simulink library "wt_blockset_v3"  (Simulink 6.0)
settings: Solver=ode45  SolverMode=SingleTasking  StartTime=0.0  StopTime=10.0  RelTol=1e-3
undefined symbols (not defined in the file): f1, get, j, Kmode, Type, u0
libraries: simulink_extras x12, simulink3 x5, simulink x4, dspinverses x1, dspmtrx3 x1, dspsnks4 x1
(part 7 of 7)

== system wt_blockset_v3/Power Converters/Average SVM Strategy/3rd quadrant/Sector 4 ==
  note: Sector 4
  vd : Inport  Port=1  LatchInput=off
  vq : Inport  Port=2  LatchInput=off
  Action Port : ActionPort  InitializeStates=reset
  Constant : Constant  Value=0.5
  Mux : Mux  Inputs=3
  Mux1 : Mux  Inputs=3
  Mux2 : Mux  Inputs=3
  Mux3 : Mux  Inputs=2
  Sum : Sum  Inputs=-+-  SaturateOnIntegerOverflow=on
  T0_pr : Fcn  Expr=(u(2)<=0)*0+(u(2)>0)*u(2)
  T1_pr : Fcn  Expr=(u(2)<=0)*(0.5*u(1)/(u(1)+u(3)))+(u(2)>0)*u(1)
  T2_pr : Fcn  Expr=(u(2)<=0)*(0.5*u(3)/(u(1)+u(3)))+(u(2)>0)*u(3)
  T_1 : Fcn  Expr=0.5*(-u(1)+abs(u(2))/sqrt(3))
  T_2 : Fcn  Expr=0.5*(u(1)+abs(u(2))/sqrt(3))
  duty_A : Fcn  Expr=1-(u(3)+2*u(1))
  duty_B : Fcn  Expr=u(3)
  duty_C : Fcn  Expr=1-u(3)
  duty_ABC : Outport  OutputWhenDisabled=reset  InitialOutput=[0 0 0]
  wires:
  Sum/1 -> Mux1/2
  Constant/1 -> Sum/2
  T_1/1 -> Sum/1, Mux1/1
  T_2/1 -> Mux1/3, Sum/3
  Mux1/1 -> T1_pr/1, T2_pr/1, T0_pr/1
  T0_pr/1 -> [T0]
  T1_pr/1 -> [T1]
  T2_pr/1 -> [T2]
  [T1] -> Mux2/1
  [T2] -> Mux2/2
  [T0] -> Mux2/3
  Mux/1 -> duty_ABC/1
  Mux2/1 -> duty_A/1, duty_B/1, duty_C/1
  duty_A/1 -> Mux/1
  Mux3/1 -> T_1/1, T_2/1
  vq/1 -> Mux3/2
  vd/1 -> Mux3/1
  duty_B/1 -> Mux/2
  duty_C/1 -> Mux/3

== system wt_blockset_v3/Power Converters/Average SVM Strategy/4th quadrant/Sector 4 ==
  note: Sector 4
  vd : Inport  Port=1  LatchInput=off
  vq : Inport  Port=2  LatchInput=off
  Action Port : ActionPort  InitializeStates=reset
  Constant : Constant  Value=0.5
  Mux : Mux  Inputs=3
  Mux1 : Mux  Inputs=3
  Mux2 : Mux  Inputs=3
  Mux3 : Mux  Inputs=2
  Sum : Sum  Inputs=-+-  SaturateOnIntegerOverflow=on
  T0_pr : Fcn  Expr=(u(2)<=0)*0+(u(2)>0)*u(2)
  T1_pr : Fcn  Expr=(u(2)<=0)*(0.5*u(1)/(u(1)+u(3)))+(u(2)>0)*u(1)
  T2_pr : Fcn  Expr=(u(2)<=0)*(0.5*u(3)/(u(1)+u(3)))+(u(2)>0)*u(3)
  T_1 : Fcn  Expr=0.5*(-u(1)+abs(u(2))/sqrt(3))
  T_2 : Fcn  Expr=0.5*(u(1)+abs(u(2))/sqrt(3))
  duty_A : Fcn  Expr=1-(u(3)+2*u(1))
  duty_B : Fcn  Expr=u(3)
  duty_C : Fcn  Expr=1-u(3)
  duty_ABC : Outport  OutputWhenDisabled=reset  InitialOutput=[0 0 0]
  wires:
  duty_C/1 -> Mux/3
  duty_B/1 -> Mux/2
  vd/1 -> Mux3/1
  vq/1 -> Mux3/2
  Mux3/1 -> T_2/1, T_1/1
  duty_A/1 -> Mux/1
  Mux2/1 -> duty_C/1, duty_B/1, duty_A/1
  Mux/1 -> duty_ABC/1
  [T0] -> Mux2/3
  [T2] -> Mux2/2
  [T1] -> Mux2/1
  T0_pr/1 -> [T0]
  T2_pr/1 -> [T2]
  T1_pr/1 -> [T1]
  Mux1/1 -> T0_pr/1, T2_pr/1, T1_pr/1
  T_2/1 -> Sum/3, Mux1/3
  T_1/1 -> Mux1/1, Sum/1
  Constant/1 -> Sum/2
  Sum/1 -> Mux1/2

== system wt_blockset_v3/Power Converters/Average SVM Strategy/4th quadrant/Sector 5 ==
  note: Sector 5
  vd : Inport  Port=1  LatchInput=off
  vq : Inport  Port=2  LatchInput=off
  Action Port : ActionPort  InitializeStates=reset
  Constant : Constant  Value=0.5
  Mux : Mux  Inputs=3
  Mux1 : Mux  Inputs=3
  Mux2 : Mux  Inputs=3
  Mux3 : Mux  Inputs=2
  Sum : Sum  Inputs=-+-  SaturateOnIntegerOverflow=on
  T0_pr : Fcn  Expr=(u(2)<=0)*0+(u(2)>0)*u(2)
  T1_pr : Fcn  Expr=(u(2)<=0)*(0.5*u(1)/(u(1)+u(3)))+(u(2)>0)*u(1)
  T2_pr : Fcn  Expr=(u(2)<=0)*(0.5*u(3)/(u(1)+u(3)))+(u(2)>0)*u(3)
  T_1 : Fcn  Expr=0.5*((u(1))-abs(u(2))/sqrt(3))
  T_2 : Fcn  Expr=abs(u(2))/sqrt(3)
  duty_A : Fcn  Expr=1-u(3)
  duty_B : Fcn  Expr=u(3)
  duty_C : Fcn  Expr=1-(u(3)+2*u(1))
  duty_ABC : Outport  OutputWhenDisabled=reset  InitialOutput=[0 0 0]
  wires:
  vd/1 -> Mux3/1
  vq/1 -> Mux3/2
  Constant/1 -> Sum/2
  Sum/1 -> Mux1/2
  T1_pr/1 -> [T1]
  T2_pr/1 -> [T2]
  T0_pr/1 -> [T0]
  Mux1/1 -> T1_pr/1, T2_pr/1, T0_pr/1
  [T1] -> Mux2/1
  [T2] -> Mux2/2
  [T0] -> Mux2/3
  Mux/1 -> duty_ABC/1
  T_2/1 -> Mux1/3, Sum/3
  T_1/1 -> Mux1/1, Sum/1
  Mux3/1 -> T_1/1, T_2/1
  duty_A/1 -> Mux/1
  duty_B/1 -> Mux/2
  duty_C/1 -> Mux/3
  Mux2/1 -> duty_B/1, duty_A/1, duty_C/1

== system wt_blockset_v3/Power Converters/Soft-Starter/S-R flip flop/S-R Flip-Flop1 ==
  S : Inport  Port=1  LatchInput=off
  R : Inport  Port=2  LatchInput=off
  Demux : Demux  Outputs=2
  Logic : CombinatorialLogic  TruthTable=[0 1;1 0;0 1;0 1;1 0;1 0;0 0;0 0]
  Memory : Memory  Orientation=left  X0=initial_condition  InheritSampleTime=on
  Mux : Mux  Inputs=3
  Q : Outport  InitialOutput=0
  !Q : Outport  Port=2  InitialOutput=1
  wires:
  Memory/1 -> Mux/3
  Mux/1 -> Logic/1
  Logic/1 -> Demux/1
  Demux/2 -> !Q/1
  Demux/1 -> Q/1, Memory/1
  S/1 -> Mux/1
  R/1 -> Mux/2

== system wt_blockset_v3/Power Converters/Soft-Starter/S-R flip flop/S-R Flip-Flop2 ==
  S : Inport  Port=1  LatchInput=off
  R : Inport  Port=2  LatchInput=off
  Demux : Demux  Outputs=2
  Logic : CombinatorialLogic  TruthTable=[0 1;1 0;0 1;0 1;1 0;1 0;0 0;0 0]
  Memory : Memory  Orientation=left  X0=initial_condition  InheritSampleTime=on
  Mux : Mux  Inputs=3
  Q : Outport  InitialOutput=0
  !Q : Outport  Port=2  InitialOutput=1
  wires:
  Memory/1 -> Mux/3
  Mux/1 -> Logic/1
  Logic/1 -> Demux/1
  Demux/2 -> !Q/1
  Demux/1 -> Q/1, Memory/1
  S/1 -> Mux/1
  R/1 -> Mux/2

== system wt_blockset_v3/Power Converters/Soft-Starter/S-R flip flop/S-R Flip-Flop3 ==
  S : Inport  Port=1  LatchInput=off
  R : Inport  Port=2  LatchInput=off
  Demux : Demux  Outputs=2
  Logic : CombinatorialLogic  TruthTable=[0 1;1 0;0 1;0 1;1 0;1 0;0 0;0 0]
  Memory : Memory  Orientation=left  X0=initial_condition  InheritSampleTime=on
  Mux : Mux  Inputs=3
  Q : Outport  InitialOutput=0
  !Q : Outport  Port=2  InitialOutput=1
  wires:
  Memory/1 -> Mux/3
  Mux/1 -> Logic/1
  Logic/1 -> Demux/1
  Demux/2 -> !Q/1
  Demux/1 -> Q/1, Memory/1
  S/1 -> Mux/1
  R/1 -> Mux/2

== system wt_blockset_v3/Power Converters/Soft-Starter/S-R flip flop/S-R Flip-Flop4 ==
  S : Inport  Port=1  LatchInput=off
  R : Inport  Port=2  LatchInput=off
  Demux : Demux  Outputs=2
  Logic : CombinatorialLogic  TruthTable=[0 1;1 0;0 1;0 1;1 0;1 0;0 0;0 0]
  Memory : Memory  Orientation=left  X0=initial_condition  InheritSampleTime=on
  Mux : Mux  Inputs=3
  Q : Outport  InitialOutput=0
  !Q : Outport  Port=2  InitialOutput=1
  wires:
  Memory/1 -> Mux/3
  Mux/1 -> Logic/1
  Logic/1 -> Demux/1
  Demux/2 -> !Q/1
  Demux/1 -> Q/1, Memory/1
  S/1 -> Mux/1
  R/1 -> Mux/2

== system wt_blockset_v3/Power Converters/Soft-Starter/S-R flip flop/S-R Flip-Flop5 ==
  S : Inport  Port=1  LatchInput=off
  R : Inport  Port=2  LatchInput=off
  Demux : Demux  Outputs=2
  Logic : CombinatorialLogic  TruthTable=[0 1;1 0;0 1;0 1;1 0;1 0;0 0;0 0]
  Memory : Memory  Orientation=left  X0=initial_condition  InheritSampleTime=on
  Mux : Mux  Inputs=3
  Q : Outport  InitialOutput=0
  !Q : Outport  Port=2  InitialOutput=1
  wires:
  Memory/1 -> Mux/3
  Mux/1 -> Logic/1
  Logic/1 -> Demux/1
  Demux/2 -> !Q/1
  Demux/1 -> Q/1, Memory/1
  S/1 -> Mux/1
  R/1 -> Mux/2

== system wt_blockset_v3/Power Converters/Soft-Starter/S-R flip flop/S-R Flip-Flop6 ==
  S : Inport  Port=1  LatchInput=off
  R : Inport  Port=2  LatchInput=off
  Demux : Demux  Outputs=2
  Logic : CombinatorialLogic  TruthTable=[0 1;1 0;0 1;0 1;1 0;1 0;0 0;0 0]
  Memory : Memory  Orientation=left  X0=initial_condition  InheritSampleTime=on
  Mux : Mux  Inputs=3
  Q : Outport  InitialOutput=0
  !Q : Outport  Port=2  InitialOutput=1
  wires:
  Memory/1 -> Mux/3
  Mux/1 -> Logic/1
  Logic/1 -> Demux/1
  Demux/2 -> !Q/1
  Demux/1 -> Q/1, Memory/1
  S/1 -> Mux/1
  R/1 -> Mux/2

== system wt_blockset_v3/Power Converters/Soft-Starter/S-R flip flop1/S-R Flip-Flop1 ==
  S : Inport  Port=1  LatchInput=off
  R : Inport  Port=2  LatchInput=off
  Demux : Demux  Outputs=2
  Logic : CombinatorialLogic  TruthTable=[0 1;1 0;0 1;0 1;1 0;1 0;0 0;0 0]
  Memory : Memory  Orientation=left  X0=initial_condition  InheritSampleTime=on
  Mux : Mux  Inputs=3
  Q : Outport  InitialOutput=0
  !Q : Outport  Port=2  InitialOutput=1
  wires:
  R/1 -> Mux/2
  S/1 -> Mux/1
  Demux/1 -> Memory/1, Q/1
  Demux/2 -> !Q/1
  Logic/1 -> Demux/1
  Mux/1 -> Logic/1
  Memory/1 -> Mux/3

== system wt_blockset_v3/Power Converters/Soft-Starter/S-R flip flop1/S-R Flip-Flop2 ==
  S : Inport  Port=1  LatchInput=off
  R : Inport  Port=2  LatchInput=off
  Demux : Demux  Outputs=2
  Logic : CombinatorialLogic  TruthTable=[0 1;1 0;0 1;0 1;1 0;1 0;0 0;0 0]
  Memory : Memory  Orientation=left  X0=initial_condition  InheritSampleTime=on
  Mux : Mux  Inputs=3
  Q : Outport  InitialOutput=0
  !Q : Outport  Port=2  InitialOutput=1
  wires:
  Memory/1 -> Mux/3
  Mux/1 -> Logic/1
  Logic/1 -> Demux/1
  Demux/2 -> !Q/1
  Demux/1 -> Q/1, Memory/1
  S/1 -> Mux/1
  R/1 -> Mux/2

== system wt_blockset_v3/Power Converters/Soft-Starter/S-R flip flop1/S-R Flip-Flop3 ==
  S : Inport  Port=1  LatchInput=off
  R : Inport  Port=2  LatchInput=off
  Demux : Demux  Outputs=2
  Logic : CombinatorialLogic  TruthTable=[0 1;1 0;0 1;0 1;1 0;1 0;0 0;0 0]
  Memory : Memory  Orientation=left  X0=initial_condition  InheritSampleTime=on
  Mux : Mux  Inputs=3
  Q : Outport  InitialOutput=0
  !Q : Outport  Port=2  InitialOutput=1
  wires:
  Memory/1 -> Mux/3
  Mux/1 -> Logic/1
  Logic/1 -> Demux/1
  Demux/2 -> !Q/1
  Demux/1 -> Q/1, Memory/1
  S/1 -> Mux/1
  R/1 -> Mux/2

== system wt_blockset_v3/Power Converters/Soft-Starter/S-R flip flop1/S-R Flip-Flop4 ==
  S : Inport  Port=1  LatchInput=off
  R : Inport  Port=2  LatchInput=off
  Demux : Demux  Outputs=2
  Logic : CombinatorialLogic  TruthTable=[0 1;1 0;0 1;0 1;1 0;1 0;0 0;0 0]
  Memory : Memory  Orientation=left  X0=initial_condition  InheritSampleTime=on
  Mux : Mux  Inputs=3
  Q : Outport  InitialOutput=0
  !Q : Outport  Port=2  InitialOutput=1
  wires:
  Memory/1 -> Mux/3
  Mux/1 -> Logic/1
  Logic/1 -> Demux/1
  Demux/2 -> !Q/1
  Demux/1 -> Q/1, Memory/1
  S/1 -> Mux/1
  R/1 -> Mux/2

== system wt_blockset_v3/Power Converters/Soft-Starter/S-R flip flop1/S-R Flip-Flop5 ==
  S : Inport  Port=1  LatchInput=off
  R : Inport  Port=2  LatchInput=off
  Demux : Demux  Outputs=2
  Logic : CombinatorialLogic  TruthTable=[0 1;1 0;0 1;0 1;1 0;1 0;0 0;0 0]
  Memory : Memory  Orientation=left  X0=initial_condition  InheritSampleTime=on
  Mux : Mux  Inputs=3
  Q : Outport  InitialOutput=0
  !Q : Outport  Port=2  InitialOutput=1
  wires:
  Memory/1 -> Mux/3
  Mux/1 -> Logic/1
  Logic/1 -> Demux/1
  Demux/2 -> !Q/1
  Demux/1 -> Q/1, Memory/1
  S/1 -> Mux/1
  R/1 -> Mux/2

== system wt_blockset_v3/Power Converters/Soft-Starter/S-R flip flop1/S-R Flip-Flop6 ==
  S : Inport  Port=1  LatchInput=off
  R : Inport  Port=2  LatchInput=off
  Demux : Demux  Outputs=2
  Logic : CombinatorialLogic  TruthTable=[0 1;1 0;0 1;0 1;1 0;1 0;0 0;0 0]
  Memory : Memory  Orientation=left  X0=initial_condition  InheritSampleTime=on
  Mux : Mux  Inputs=3
  Q : Outport  InitialOutput=0
  !Q : Outport  Port=2  InitialOutput=1
  wires:
  Memory/1 -> Mux/3
  Mux/1 -> Logic/1
  Logic/1 -> Demux/1
  Demux/2 -> !Q/1
  Demux/1 -> Q/1, Memory/1
  S/1 -> Mux/1
  R/1 -> Mux/2

== system wt_blockset_v3/Power Converters/Switching PWM Strategy/capcom/Vtri1 ==
  Constant1 : Constant
  Constant2 : Constant
  Constant3 : Constant  Value=0
  Data Type Conversion : DataTypeConversion  SaturateOnIntegerOverflow=on  RndMeth=Zero
  Fcn : Fcn  Expr=-u(1)*2+1
  Gain : Gain  Gain=fsw2  SaturateOnIntegerOverflow=on
  Gain1 : Gain  Gain=2*fsw2  SaturateOnIntegerOverflow=on
  IC : InitialCondition  Value=1.5
  Integrator : Integrator  ExternalReset=rising  InitialConditionSource=external  InitialCondition=1.5
  Integrator1 : Integrator  ExternalReset=rising
  Pulse Generator : DiscretePulseGenerator  PulseType=Time based  Period=2/fsw2  PulseWidth=50  PhaseDelay=0.5/fsw2
  Pulse Generator1 : DiscretePulseGenerator  PulseType=Time based  Period=2/fsw2  PulseWidth=50
  Relational Operator : RelationalOperator  InputSameDT=on
  Vtri : Outport  InitialOutput=0
  wires:
  Integrator1/1 -> Vtri/1
  Pulse Generator/1 -> Integrator/2
  Constant2/1 -> Gain/1
  Fcn/1 -> Gain1/1
  Relational Operator/1 -> Data Type Conversion/1
  Integrator/1 -> Relational Operator/1
  IC/1 -> Integrator/3
  Constant3/1 -> IC/1
  Pulse Generator1/1 -> Integrator1/2
  Gain1/1 -> Integrator1/1
  Gain/1 -> Integrator/1
  Constant1/1 -> Relational Operator/2
  Data Type Conversion/1 -> Fcn/1

== system wt_blockset_v3/Power Converters/Switching PWM Strategy/capcom/pulses ==
  In1 : Inport  Port=1  LatchInput=off
  Constant : Constant  Value=0
  Data Type Conversion : DataTypeConversion  OutDataTypeMode=double  SaturateOnIntegerOverflow=on  RndMeth=Zero
  Hit  Crossing : HitCross  ShowOutputPort=off
  IC : InitialCondition  Value=0
  Relational Operator : RelationalOperator  InputSameDT=on
  Out1 : Outport  InitialOutput=0
  wires:
  Relational Operator/1 -> Data Type Conversion/1
  In1/1 -> Relational Operator/1
  Constant/1 -> Relational Operator/2
  IC/1 -> Out1/1
  Data Type Conversion/1 -> Hit  Crossing/1, IC/1

== system wt_blockset_v3/Power Converters/Switching SVM Strategy/1st quadrant/Sector 0 ==
  note: Sector 0
  vd : Inport  Port=1  LatchInput=off
  vq : Inport  Port=2  LatchInput=off
  Action Port : ActionPort  InitializeStates=reset
  Constant : Constant  Value=0.5
  Mux : Mux  Inputs=3
  Mux1 : Mux  Inputs=3
  Mux2 : Mux  Inputs=3
  Mux3 : Mux  Inputs=2
  Sum : Sum  Inputs=-+-  SaturateOnIntegerOverflow=on
  T0_pr : Fcn  Expr=(u(2)<=0)*0+(u(2)>0)*u(2)
  T1_pr : Fcn  Expr=(u(2)<=0)*(0.5*u(1)/(u(1)+u(3)))+(u(2)>0)*u(1)
  T2_pr : Fcn  Expr=(u(2)<=0)*(0.5*u(3)/(u(1)+u(3)))+(u(2)>0)*u(3)
  T_1 : Fcn  Expr=0.5*(u(1)-u(2)/sqrt(3))
  T_2 : Fcn  Expr=u(2)/sqrt(3)
  duty_A : Fcn  Expr=1-u(3)
  duty_B : Fcn  Expr=1-(u(3)+2*u(1))
  duty_C : Fcn  Expr=u(3)
  duty_ABC : Outport  OutputWhenDisabled=reset  InitialOutput=[0 0 0]
  wires:
  T_2/1 -> Sum/3, Mux1/3
  T_1/1 -> Sum/1, Mux1/1
  Constant/1 -> Sum/2
  Sum/1 -> Mux1/2
  T1_pr/1 -> [T1]
  T2_pr/1 -> [T2]
  T0_pr/1 -> [T0]
  Mux1/1 -> T1_pr/1, T2_pr/1, T0_pr/1
  [T1] -> Mux2/1
  [T2] -> Mux2/2
  [T0] -> Mux2/3
  Mux2/1 -> duty_B/1, duty_A/1, duty_C/1
  duty_A/1 -> Mux/1
  duty_B/1 -> Mux/2
  duty_C/1 -> Mux/3
  Mux/1 -> duty_ABC/1
  Mux3/1 -> T_1/1, T_2/1
  vd/1 -> Mux3/1
  vq/1 -> Mux3/2

== system wt_blockset_v3/Power Converters/Switching SVM Strategy/1st quadrant/Sector 1 ==
  note: Sector 1
  vd : Inport  Port=1  LatchInput=off
  vq : Inport  Port=2  LatchInput=off
  Action Port : ActionPort  InitializeStates=reset
  Constant : Constant  Value=0.5
  Mux : Mux  Inputs=3
  Mux1 : Mux  Inputs=3
  Mux2 : Mux  Inputs=3
  Mux3 : Mux  Inputs=2
  Sum : Sum  Inputs=-+-  SaturateOnIntegerOverflow=on
  T0_pr : Fcn  Expr=(u(2)<=0)*0+(u(2)>0)*u(2)
  T1_pr : Fcn  Expr=(u(2)<=0)*(0.5*u(1)/(u(1)+u(3)))+(u(2)>0)*u(1)
  T2_pr : Fcn  Expr=(u(2)<=0)*(0.5*u(3)/(u(1)+u(3)))+(u(2)>0)*u(3)
  T_1 : Fcn  Expr=0.5*(-u(1)+u(2)/sqrt(3))
  T_2 : Fcn  Expr=0.5*(+u(1)+u(2)/sqrt(3))
  duty_A : Fcn  Expr=1-(u(3)+2*u(1))
  duty_B : Fcn  Expr=1-u(3)
  duty_C : Fcn  Expr=u(3)
  duty_ABC : Outport  OutputWhenDisabled=reset  InitialOutput=[0 0 0]
  wires:
  Sum/1 -> Mux1/2
  Constant/1 -> Sum/2
  T_1/1 -> Sum/1, Mux1/1
  T_2/1 -> Mux1/3, Sum/3
  Mux1/1 -> T1_pr/1, T2_pr/1, T0_pr/1
  [T1] -> Mux2/1
  [T2] -> Mux2/2
  [T0] -> Mux2/3
  Mux/1 -> duty_ABC/1
  Mux2/1 -> duty_B/1, duty_A/1, duty_C/1
  duty_B/1 -> Mux/2
  duty_A/1 -> Mux/1
  duty_C/1 -> Mux/3
  Mux3/1 -> T_1/1, T_2/1
  vq/1 -> Mux3/2
  vd/1 -> Mux3/1
  T1_pr/1 -> [T1]
  T2_pr/1 -> [T2]
  T0_pr/1 -> [T0]

== system wt_blockset_v3/Power Converters/Switching SVM Strategy/2nd quadrant/Sector 1 ==
  note: Sector 1
  vd : Inport  Port=1  LatchInput=off
  vq : Inport  Port=2  LatchInput=off
  Action Port : ActionPort  InitializeStates=reset
  Constant : Constant  Value=0.5
  Mux : Mux  Inputs=3
  Mux1 : Mux  Inputs=3
  Mux2 : Mux  Inputs=3
  Mux3 : Mux  Inputs=2
  Sum : Sum  Inputs=-+-  SaturateOnIntegerOverflow=on
  T0_pr : Fcn  Expr=(u(2)<=0)*0+(u(2)>0)*u(2)
  T1_pr : Fcn  Expr=(u(2)<=0)*(0.5*u(1)/(u(1)+u(3)))+(u(2)>0)*u(1)
  T2_pr : Fcn  Expr=(u(2)<=0)*(0.5*u(3)/(u(1)+u(3)))+(u(2)>0)*u(3)
  T_1 : Fcn  Expr=0.5*(-u(1)+u(2)/sqrt(3))
  T_2 : Fcn  Expr=0.5*(+u(1)+u(2)/sqrt(3))
  duty_A : Fcn  Expr=1-(u(3)+2*u(1))
  duty_B : Fcn  Expr=1-u(3)
  duty_C : Fcn  Expr=u(3)
  duty_ABC : Outport  OutputWhenDisabled=reset  InitialOutput=[0 0 0]
  wires:
  Sum/1 -> Mux1/2
  Constant/1 -> Sum/2
  T_1/1 -> Sum/1, Mux1/1
  T_2/1 -> Mux1/3, Sum/3
  Mux1/1 -> T1_pr/1, T2_pr/1, T0_pr/1
  [T1] -> Mux2/1
  [T2] -> Mux2/2
  [T0] -> Mux2/3
  Mux/1 -> duty_ABC/1
  Mux2/1 -> duty_B/1, duty_A/1, duty_C/1
  duty_B/1 -> Mux/2
  duty_A/1 -> Mux/1
  duty_C/1 -> Mux/3
  Mux3/1 -> T_1/1, T_2/1
  vq/1 -> Mux3/2
  vd/1 -> Mux3/1
  T1_pr/1 -> [T1]
  T2_pr/1 -> [T2]
  T0_pr/1 -> [T0]

== system wt_blockset_v3/Power Converters/Switching SVM Strategy/2nd quadrant/Sector 2 ==
  note: Sector 2
  vd : Inport  Port=1  LatchInput=off
  vq : Inport  Port=2  LatchInput=off
  Action Port : ActionPort  InitializeStates=reset
  Constant : Constant  Value=0.5
  Mux : Mux  Inputs=3
  Mux1 : Mux  Inputs=3
  Mux2 : Mux  Inputs=3
  Mux3 : Mux  Inputs=2
  Sum : Sum  Inputs=-+-  SaturateOnIntegerOverflow=on
  T0_pr : Fcn  Expr=(u(2)<=0)*0+(u(2)>0)*u(2)
  T1_pr : Fcn  Expr=(u(2)<=0)*(0.5*u(1)/(u(1)+u(3)))+(u(2)>0)*u(1)
  T2_pr : Fcn  Expr=(u(2)<=0)*(0.5*u(3)/(u(1)+u(3)))+(u(2)>0)*u(3)
  T_ : Fcn  Expr=0.5*(abs(u(1))-u(2)/sqrt(3))
  T_1 : Fcn  Expr=u(2)/sqrt(3)
  duty_A : Fcn  Expr=u(3)
  duty_B : Fcn  Expr=1-u(3)
  duty_C : Fcn  Expr=1-(u(3)+2*u(1))
  duty_ABC : Outport  OutputWhenDisabled=reset  InitialOutput=[0 0 0]
  wires:
  Mux/1 -> duty_ABC/1
  [T0] -> Mux2/3
  [T2] -> Mux2/2
  [T1] -> Mux2/1
  Mux1/1 -> T0_pr/1, T2_pr/1, T1_pr/1
  Sum/1 -> Mux1/2
  Constant/1 -> Sum/2
  vq/1 -> Mux3/2
  vd/1 -> Mux3/1
  Mux3/1 -> T_1/1, T_/1
  T_1/1 -> Mux1/1, Sum/1
  T_/1 -> Mux1/3, Sum/3
  duty_B/1 -> Mux/2
  duty_A/1 -> Mux/1
  duty_C/1 -> Mux/3
  Mux2/1 -> duty_B/1, duty_A/1, duty_C/1
  T1_pr/1 -> [T1]
  T2_pr/1 -> [T2]
  T0_pr/1 -> [T0]

== system wt_blockset_v3/Power Converters/Switching SVM Strategy/3rd quadrant/Sector 3 ==
  note: Sector 2
  vd : Inport  Port=1  LatchInput=off
  vq : Inport  Port=2  LatchInput=off
  Action Port : ActionPort  InitializeStates=reset
  Constant : Constant  Value=0.5
  Mux : Mux  Inputs=3
  Mux1 : Mux  Inputs=3
  Mux2 : Mux  Inputs=3
  Mux3 : Mux  Inputs=2
  Sum : Sum  Inputs=-+-  SaturateOnIntegerOverflow=on
  T0_pr : Fcn  Expr=(u(2)<=0)*0+(u(2)>0)*u(2)
  T1_pr : Fcn  Expr=(u(2)<=0)*(0.5*u(1)/(u(1)+u(3)))+(u(2)>0)*u(1)
  T2_pr : Fcn  Expr=(u(2)<=0)*(0.5*u(3)/(u(1)+u(3)))+(u(2)>0)*u(3)
  T_ : Fcn  Expr=0.5*(abs(u(1))-abs(u(2))/sqrt(3))
  T_1 : Fcn  Expr=abs(u(2))/sqrt(3)
  duty_A : Fcn  Expr=u(3)
  duty_B : Fcn  Expr=1-(u(3)+2*u(1))
  duty_C : Fcn  Expr=1-u(3)
  duty_ABC : Outport  OutputWhenDisabled=reset  InitialOutput=[0 0 0]
  wires:
  Mux/1 -> duty_ABC/1
  [T0] -> Mux2/3
  [T2] -> Mux2/2
  [T1] -> Mux2/1
  Mux1/1 -> T0_pr/1, T2_pr/1, T1_pr/1
  Sum/1 -> Mux1/2
  Constant/1 -> Sum/2
  vq/1 -> Mux3/2
  vd/1 -> Mux3/1
  Mux3/1 -> T_1/1, T_/1
  T_1/1 -> Mux1/1, Sum/1
  T_/1 -> Mux1/3, Sum/3
  duty_A/1 -> Mux/1
  Mux2/1 -> duty_A/1, duty_B/1, duty_C/1
  duty_B/1 -> Mux/2
  duty_C/1 -> Mux/3
  T1_pr/1 -> [T1]
  T2_pr/1 -> [T2]
  T0_pr/1 -> [T0]

== system wt_blockset_v3/Power Converters/Switching SVM Strategy/3rd quadrant/Sector 4 ==
  note: Sector 4
  vd : Inport  Port=1  LatchInput=off
  vq : Inport  Port=2  LatchInput=off
  Action Port : ActionPort  InitializeStates=reset
  Constant : Constant  Value=0.5
  Mux : Mux  Inputs=3
  Mux1 : Mux  Inputs=3
  Mux2 : Mux  Inputs=3
  Mux3 : Mux  Inputs=2
  Sum : Sum  Inputs=-+-  SaturateOnIntegerOverflow=on
  T0_pr : Fcn  Expr=(u(2)<=0)*0+(u(2)>0)*u(2)
  T1_pr : Fcn  Expr=(u(2)<=0)*(0.5*u(1)/(u(1)+u(3)))+(u(2)>0)*u(1)
  T2_pr : Fcn  Expr=(u(2)<=0)*(0.5*u(3)/(u(1)+u(3)))+(u(2)>0)*u(3)
  T_1 : Fcn  Expr=0.5*(-u(1)+abs(u(2))/sqrt(3))
  T_2 : Fcn  Expr=0.5*(u(1)+abs(u(2))/sqrt(3))
  duty_A : Fcn  Expr=1-(u(3)+2*u(1))
  duty_B : Fcn  Expr=u(3)
  duty_C : Fcn  Expr=1-u(3)
  duty_ABC : Outport  OutputWhenDisabled=reset  InitialOutput=[0 0 0]
  wires:
  Sum/1 -> Mux1/2
  Constant/1 -> Sum/2
  T_1/1 -> Sum/1, Mux1/1
  T_2/1 -> Mux1/3, Sum/3
  Mux1/1 -> T1_pr/1, T2_pr/1, T0_pr/1
  [T1] -> Mux2/1
  [T2] -> Mux2/2
  [T0] -> Mux2/3
  Mux/1 -> duty_ABC/1
  Mux2/1 -> duty_A/1, duty_B/1, duty_C/1
  duty_A/1 -> Mux/1
  Mux3/1 -> T_1/1, T_2/1
  vq/1 -> Mux3/2
  vd/1 -> Mux3/1
  duty_B/1 -> Mux/2
  duty_C/1 -> Mux/3
  T1_pr/1 -> [T1]
  T2_pr/1 -> [T2]
  T0_pr/1 -> [T0]

== system wt_blockset_v3/Power Converters/Switching SVM Strategy/4th quadrant/Sector 4 ==
  note: Sector 4
  vd : Inport  Port=1  LatchInput=off
  vq : Inport  Port=2  LatchInput=off
  Action Port : ActionPort  InitializeStates=reset
  Constant : Constant  Value=0.5
  Mux : Mux  Inputs=3
  Mux1 : Mux  Inputs=3
  Mux2 : Mux  Inputs=3
  Mux3 : Mux  Inputs=2
  Sum : Sum  Inputs=-+-  SaturateOnIntegerOverflow=on
  T0_pr : Fcn  Expr=(u(2)<=0)*0+(u(2)>0)*u(2)
  T1_pr : Fcn  Expr=(u(2)<=0)*(0.5*u(1)/(u(1)+u(3)))+(u(2)>0)*u(1)
  T2_pr : Fcn  Expr=(u(2)<=0)*(0.5*u(3)/(u(1)+u(3)))+(u(2)>0)*u(3)
  T_1 : Fcn  Expr=0.5*(-u(1)+abs(u(2))/sqrt(3))
  T_2 : Fcn  Expr=0.5*(u(1)+abs(u(2))/sqrt(3))
  duty_A : Fcn  Expr=1-(u(3)+2*u(1))
  duty_B : Fcn  Expr=u(3)
  duty_C : Fcn  Expr=1-u(3)
  duty_ABC : Outport  OutputWhenDisabled=reset  InitialOutput=[0 0 0]
  wires:
  duty_C/1 -> Mux/3
  duty_B/1 -> Mux/2
  vd/1 -> Mux3/1
  vq/1 -> Mux3/2
  Mux3/1 -> T_2/1, T_1/1
  duty_A/1 -> Mux/1
  Mux2/1 -> duty_C/1, duty_B/1, duty_A/1
  Mux/1 -> duty_ABC/1
  [T0] -> Mux2/3
  [T2] -> Mux2/2
  [T1] -> Mux2/1
  Mux1/1 -> T0_pr/1, T2_pr/1, T1_pr/1
  T_2/1 -> Sum/3, Mux1/3
  T_1/1 -> Mux1/1, Sum/1
  Constant/1 -> Sum/2
  Sum/1 -> Mux1/2
  T1_pr/1 -> [T1]
  T2_pr/1 -> [T2]
  T0_pr/1 -> [T0]

== system wt_blockset_v3/Power Converters/Switching SVM Strategy/4th quadrant/Sector 5 ==
  note: Sector 5
  vd : Inport  Port=1  LatchInput=off
  vq : Inport  Port=2  LatchInput=off
  Action Port : ActionPort  InitializeStates=reset
  Constant : Constant  Value=0.5
  Mux : Mux  Inputs=3
  Mux1 : Mux  Inputs=3
  Mux2 : Mux  Inputs=3
  Mux3 : Mux  Inputs=2
  Sum : Sum  Inputs=-+-  SaturateOnIntegerOverflow=on
  T0_pr : Fcn  Expr=(u(2)<=0)*0+(u(2)>0)*u(2)
  T1_pr : Fcn  Expr=(u(2)<=0)*(0.5*u(1)/(u(1)+u(3)))+(u(2)>0)*u(1)
  T2_pr : Fcn  Expr=(u(2)<=0)*(0.5*u(3)/(u(1)+u(3)))+(u(2)>0)*u(3)
  T_1 : Fcn  Expr=0.5*((u(1))-abs(u(2))/sqrt(3))
  T_2 : Fcn  Expr=abs(u(2))/sqrt(3)
  duty_A : Fcn  Expr=1-u(3)
  duty_B : Fcn  Expr=u(3)
  duty_C : Fcn  Expr=1-(u(3)+2*u(1))
  duty_ABC : Outport  OutputWhenDisabled=reset  InitialOutput=[0 0 0]
  wires:
  vd/1 -> Mux3/1
  vq/1 -> Mux3/2
  Constant/1 -> Sum/2
  Sum/1 -> Mux1/2
  Mux1/1 -> T1_pr/1, T2_pr/1, T0_pr/1
  [T1] -> Mux2/1
  [T2] -> Mux2/2
  [T0] -> Mux2/3
  Mux/1 -> duty_ABC/1
  T_2/1 -> Mux1/3, Sum/3
  T_1/1 -> Mux1/1, Sum/1
  Mux3/1 -> T_1/1, T_2/1
  duty_A/1 -> Mux/1
  duty_B/1 -> Mux/2
  duty_C/1 -> Mux/3
  Mux2/1 -> duty_B/1, duty_A/1, duty_C/1
  T1_pr/1 -> [T1]
  T2_pr/1 -> [T2]
  T0_pr/1 -> [T0]

== system wt_blockset_v3/Electrical Machinery/Simulink Blocks  based Models/Permanent Magnet Synchronous Machine with iron losses/PMSM d-q/Iron losses resistance ==
  wr : Inport  Port=1  LatchInput=off
  Iron losses resistance : Fcn  Expr=0.0329*u[1] /(2*pi)+0.827
  Ri : Outport
  wires:
  wr/1 -> Iron losses resistance/1
  Iron losses resistance/1 -> Ri/1

== system wt_blockset_v3/Electrical Machinery/Simulink Blocks  based Models/Salient-Pole Synchronous Machine constant parameters/Mathematical model/dq / abc ==
  D : Inport  Port=1  LatchInput=off
  Q : Inport  Port=2  LatchInput=off
  theta : Inport  Port=3  LatchInput=off
  Mux : Mux  Inputs=3
  va : Fcn  Expr=u[1]*cos(u[3])-u[2]*sin(u[3])
  vb : Fcn  Expr=u[1]*cos(u[3]-2*pi/3)-u[2]*sin(u[3]-2*pi/3)
  vc : Fcn  Expr=u[1]*cos(u[3]+2*pi/3)-u[2]*sin(u[3]+2*pi/3)
  A : Outport  InitialOutput=0
  B : Outport  Port=2  InitialOutput=0
  C : Outport  Port=3  InitialOutput=0
  wires:
  va/1 -> A/1
  vb/1 -> B/1
  vc/1 -> C/1
  Mux/1 -> va/1, vb/1, vc/1
  D/1 -> Mux/1
  Q/1 -> Mux/2
  theta/1 -> Mux/3

== system wt_blockset_v3/Mechanical Components/Wind Model SB-2/3rd_Harmonic_Filter1/3rd harmonic Filter/Coefficients ==
  avg_wind : Inport  Port=1  LatchInput=off
  BD coeff : Fcn  Expr=0.2766/0.3691/(r/u(1))
  CD coeff : Fcn  Expr=0.0307/0.3691/(r/u(1))^2
  ED coeff : Fcn  Expr=1.7722/0.3691/(r/u(1))
  FD coeff : Fcn  Expr=1/0.3691/(r/u(1))^2
  BD : Outport
  CD : Outport  Port=2
  ED : Outport  Port=3
  FD : Outport  Port=4
  wires:
  avg_wind/1 -> BD coeff/1, CD coeff/1, ED coeff/1, FD coeff/1
  BD coeff/1 -> BD/1
  CD coeff/1 -> CD/1
  ED coeff/1 -> ED/1
  FD coeff/1 -> FD/1

== system wt_blockset_v3/Mechanical Components/Wind Model SB-2/3rd_Harmonic_Filter2/3rd harmonic Filter/Coefficients ==
  avg_wind : Inport  Port=1  LatchInput=off
  BD coeff : Fcn  Expr=0.2766/0.3691/(r/u(1))
  CD coeff : Fcn  Expr=0.0307/0.3691/(r/u(1))^2
  ED coeff : Fcn  Expr=1.7722/0.3691/(r/u(1))
  FD coeff : Fcn  Expr=1/0.3691/(r/u(1))^2
  BD : Outport
  CD : Outport  Port=2
  ED : Outport  Port=3
  FD : Outport  Port=4
  wires:
  FD coeff/1 -> FD/1
  ED coeff/1 -> ED/1
  CD coeff/1 -> CD/1
  BD coeff/1 -> BD/1
  avg_wind/1 -> FD coeff/1, ED coeff/1, CD coeff/1, BD coeff/1

== system wt_blockset_v3/Mechanical Components/Wind Model SB-2/Kaimal_Filter_1/Kaimal Filter/Coefficients ==
  avg_wind : Inport  Port=1  LatchInput=off
  BD coeff : Fcn  Expr=1.3653/1.3463/(L/2/pi/u(1))
  CD coeff : Fcn  Expr=0.9846/1.3463/(L/2/pi/u(1))^2
  ED coeff : Fcn  Expr=3.7593/1.3463/(L/2/pi/u(1))
  FD coeff : Fcn  Expr=1/1.3463/(L/2/pi/u(1))^2
  BD : Outport
  CD : Outport  Port=2
  ED : Outport  Port=3
  FD : Outport  Port=4
  wires:
  avg_wind/1 -> BD coeff/1, CD coeff/1, ED coeff/1, FD coeff/1
  BD coeff/1 -> BD/1
  CD coeff/1 -> CD/1
  ED coeff/1 -> ED/1
  FD coeff/1 -> FD/1

== system wt_blockset_v3/Mechanical Components/Wind Model SB-2/Kaimal_Filter_2/Kaimal Filter/Coefficients ==
  avg_wind : Inport  Port=1  LatchInput=off
  BD coeff : Fcn  Expr=1.3653/1.3463/(L/2/pi/u(1))
  CD coeff : Fcn  Expr=0.9846/1.3463/(L/2/pi/u(1))^2
  ED coeff : Fcn  Expr=3.7593/1.3463/(L/2/pi/u(1))
  FD coeff : Fcn  Expr=1/1.3463/(L/2/pi/u(1))^2
  BD : Outport
  CD : Outport  Port=2
  ED : Outport  Port=3
  FD : Outport  Port=4
  wires:
  FD coeff/1 -> FD/1
  ED coeff/1 -> ED/1
  CD coeff/1 -> CD/1
  BD coeff/1 -> BD/1
  avg_wind/1 -> FD coeff/1, ED coeff/1, CD coeff/1, BD coeff/1

== system wt_blockset_v3/Mechanical Components/Wind Model SB-2/Kaimal_Filter_3/Kaimal Filter/Coefficients ==
  avg_wind : Inport  Port=1  LatchInput=off
  BD coeff : Fcn  Expr=1.3653/1.3463/(L/2/pi/u(1))
  CD coeff : Fcn  Expr=0.9846/1.3463/(L/2/pi/u(1))^2
  ED coeff : Fcn  Expr=3.7593/1.3463/(L/2/pi/u(1))
  FD coeff : Fcn  Expr=1/1.3463/(L/2/pi/u(1))^2
  BD : Outport
  CD : Outport  Port=2
  ED : Outport  Port=3
  FD : Outport  Port=4
  wires:
  avg_wind/1 -> BD coeff/1, CD coeff/1, ED coeff/1, FD coeff/1
  BD coeff/1 -> BD/1
  CD coeff/1 -> CD/1
  ED coeff/1 -> ED/1
  FD coeff/1 -> FD/1

== system wt_blockset_v3/Mechanical Components/Wind Model SB-2/ZERO_Harmonic_Filter/ZERO harmonic Filter/Coefficients ==
  avg_wind : Inport  Port=1  LatchInput=off
  BD coeff : Fcn  Expr=4.7869/7.6823/(r/u(1))
  CD coeff : Fcn  Expr=0.9904/7.6823/(r/u(1))^2
  ED coeff : Fcn  Expr=7.3518/7.6823/(r/u(1))
  FD coeff : Fcn  Expr=1/7.6823/(r/u(1))^2
  BD : Outport
  CD : Outport  Port=2
  ED : Outport  Port=3
  FD : Outport  Port=4
  wires:
  FD coeff/1 -> FD/1
  ED coeff/1 -> ED/1
  CD coeff/1 -> CD/1
  BD coeff/1 -> BD/1
  avg_wind/1 -> FD coeff/1, ED coeff/1, CD coeff/1, BD coeff/1

== system wt_blockset_v3/Mechanical Components/Wind Model ZA-2/3rd_Harmonic_Filter1/3rd harmonic Filter/Coefficients ==
  avg_wind : Inport  Port=1  LatchInput=off
  BD coeff : Fcn  Expr=0.2766/0.3691/(r/u(1))
  CD coeff : Fcn  Expr=0.0307/0.3691/(r/u(1))^2
  ED coeff : Fcn  Expr=1.7722/0.3691/(r/u(1))
  FD coeff : Fcn  Expr=1/0.3691/(r/u(1))^2
  BD : Outport
  CD : Outport  Port=2
  ED : Outport  Port=3
  FD : Outport  Port=4
  wires:
  avg_wind/1 -> BD coeff/1, CD coeff/1, ED coeff/1, FD coeff/1
  BD coeff/1 -> BD/1
  CD coeff/1 -> CD/1
  ED coeff/1 -> ED/1
  FD coeff/1 -> FD/1

== system wt_blockset_v3/Mechanical Components/Wind Model ZA-2/3rd_Harmonic_Filter2/3rd harmonic Filter/Coefficients ==
  avg_wind : Inport  Port=1  LatchInput=off
  BD coeff : Fcn  Expr=0.2766/0.3691/(r/u(1))
  CD coeff : Fcn  Expr=0.0307/0.3691/(r/u(1))^2
  ED coeff : Fcn  Expr=1.7722/0.3691/(r/u(1))
  FD coeff : Fcn  Expr=1/0.3691/(r/u(1))^2
  BD : Outport
  CD : Outport  Port=2
  ED : Outport  Port=3
  FD : Outport  Port=4
  wires:
  FD coeff/1 -> FD/1
  ED coeff/1 -> ED/1
  CD coeff/1 -> CD/1
  BD coeff/1 -> BD/1
  avg_wind/1 -> FD coeff/1, ED coeff/1, CD coeff/1, BD coeff/1

== system wt_blockset_v3/Mechanical Components/Wind Model ZA-2/Kaimal_Filter_1/Kaimal Filter/Coefficients ==
  avg_wind : Inport  Port=1  LatchInput=off
  BD coeff : Fcn  Expr=1.3653/1.3463/(L/2/pi/u(1))
  CD coeff : Fcn  Expr=0.9846/1.3463/(L/2/pi/u(1))^2
  ED coeff : Fcn  Expr=3.7593/1.3463/(L/2/pi/u(1))
  FD coeff : Fcn  Expr=1/1.3463/(L/2/pi/u(1))^2
  BD : Outport
  CD : Outport  Port=2
  ED : Outport  Port=3
  FD : Outport  Port=4
  wires:
  avg_wind/1 -> BD coeff/1, CD coeff/1, ED coeff/1, FD coeff/1
  BD coeff/1 -> BD/1
  CD coeff/1 -> CD/1
  ED coeff/1 -> ED/1
  FD coeff/1 -> FD/1

== system wt_blockset_v3/Mechanical Components/Wind Model ZA-2/Kaimal_Filter_2/Kaimal Filter/Coefficients ==
  avg_wind : Inport  Port=1  LatchInput=off
  BD coeff : Fcn  Expr=1.3653/1.3463/(L/2/pi/u(1))
  CD coeff : Fcn  Expr=0.9846/1.3463/(L/2/pi/u(1))^2
  ED coeff : Fcn  Expr=3.7593/1.3463/(L/2/pi/u(1))
  FD coeff : Fcn  Expr=1/1.3463/(L/2/pi/u(1))^2
  BD : Outport
  CD : Outport  Port=2
  ED : Outport  Port=3
  FD : Outport  Port=4
  wires:
  FD coeff/1 -> FD/1
  ED coeff/1 -> ED/1
  CD coeff/1 -> CD/1
  BD coeff/1 -> BD/1
  avg_wind/1 -> FD coeff/1, ED coeff/1, CD coeff/1, BD coeff/1

== system wt_blockset_v3/Mechanical Components/Wind Model ZA-2/Kaimal_Filter_3/Kaimal Filter/Coefficients ==
  avg_wind : Inport  Port=1  LatchInput=off
  BD coeff : Fcn  Expr=1.3653/1.3463/(L/2/pi/u(1))
  CD coeff : Fcn  Expr=0.9846/1.3463/(L/2/pi/u(1))^2
  ED coeff : Fcn  Expr=3.7593/1.3463/(L/2/pi/u(1))
  FD coeff : Fcn  Expr=1/1.3463/(L/2/pi/u(1))^2
  BD : Outport
  CD : Outport  Port=2
  ED : Outport  Port=3
  FD : Outport  Port=4
  wires:
  avg_wind/1 -> BD coeff/1, CD coeff/1, ED coeff/1, FD coeff/1
  BD coeff/1 -> BD/1
  CD coeff/1 -> CD/1
  ED coeff/1 -> ED/1
  FD coeff/1 -> FD/1

== system wt_blockset_v3/Mechanical Components/Wind Model ZA-2/ZERO_Harmonic_Filter/ZERO harmonic Filter/Coefficients ==
  avg_wind : Inport  Port=1  LatchInput=off
  BD coeff : Fcn  Expr=4.7869/7.6823/(r/u(1))
  CD coeff : Fcn  Expr=0.9904/7.6823/(r/u(1))^2
  ED coeff : Fcn  Expr=7.3518/7.6823/(r/u(1))
  FD coeff : Fcn  Expr=1/7.6823/(r/u(1))^2
  BD : Outport
  CD : Outport  Port=2
  ED : Outport  Port=3
  FD : Outport  Port=4
  wires:
  FD coeff/1 -> FD/1
  ED coeff/1 -> ED/1
  CD coeff/1 -> CD/1
  BD coeff/1 -> BD/1
  avg_wind/1 -> FD coeff/1, ED coeff/1, CD coeff/1, BD coeff/1
